simulink model "twoDoF_I_PDandFF_assign"  (R2019b)
settings: Solver=VariableStepAuto  StartTime=0.0  StopTime=10.0  RelTol=1e-3
undefined symbols (not defined in the file): Kd, Kff, Ki, Kp, mu, Tc
libraries: DeltaBlocks x2
settings Model: Creator=Student  LastModifiedBy=Student

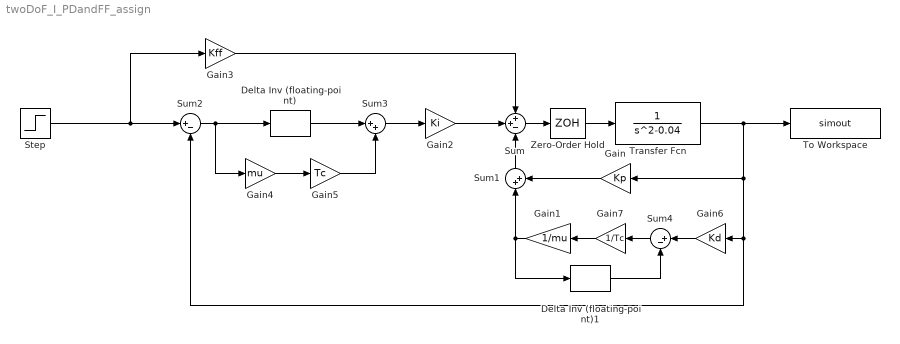
== system twoDoF_I_PDandFF_assign ==
  Delta Inv (floating-point) : DeltaBlocks/Delta Inv (floating-point)  T=Tc
  Delta Inv (floating-point)1 : DeltaBlocks/Delta Inv (floating-point)  T=Tc
  Gain : Gain  Gain=Kp
  Gain1 : Gain  Gain=1/mu
  Gain2 : Gain  Gain=Ki
  Gain3 : Gain  Gain=Kff
  Gain4 : Gain  Gain=mu
  Gain5 : Gain  Gain=Tc
  Gain6 : Gain  Gain=Kd
  Gain7 : Gain  Gain=1/Tc
  Step : Step  Time=0  SampleTime=0
  Sum : Sum  Inputs=++-
  Sum1 : Sum  Inputs=|++
  Sum2 : Sum  Inputs=|+-
  Sum3 : Sum  Inputs=|++
  Sum4 : Sum  Inputs=|+-
  To Workspace : ToWorkspace  VariableName=simout  SaveFormat=Timeseries  SampleTime=-1
  Transfer Fcn : TransferFcn  Denominator=[1 0 -0.04]
  Zero-Order Hold : ZeroOrderHold  SampleTime=Tc
  wires:
  Step/1 -> Gain3/1, Sum2/1
  Gain/1 -> Sum1/2
  Delta Inv (floating-point)/1 -> Sum3/1
  Sum2/1 -> Gain4/1, Delta Inv (floating-point)/1
  Gain2/1 -> Sum/2
  Sum1/1 -> Sum/3
  Gain3/1 -> Sum/1
  Gain4/1 -> Gain5/1
  Gain5/1 -> Sum3/2
  Sum3/1 -> Gain2/1
  Transfer Fcn/1 -> To Workspace/1, Gain/1, Gain6/1, Sum2/2
  Gain6/1 -> Sum4/1
  Delta Inv (floating-point)1/1 -> Sum4/2
  Sum4/1 -> Gain7/1
  Gain7/1 -> Gain1/1
  Gain1/1 -> Delta Inv (floating-point)1/1, Sum1/1
  Sum/1 -> Zero-Order Hold/1
  Zero-Order Hold/1 -> Transfer Fcn/1
